simulink model "simulation"  (R2019a)
settings: Solver=VariableStepAuto  StartTime=0.0  StopTime=10  RelTol=1e-3
values from neighbouring files (symbols this model uses):
  kt = sqrt(4 * ky)    [Parameters.m]
  kx = 50    [Parameters.m]
  ky = 16 / Distance^2    (= 0.04)    [Parameters.m]
libraries: simulink x5, dspsrcs4 x1
settings Model: Creator=robot  LastModifiedBy=robot
settings DebuggingCC: AlgebraicLoopMsg=none

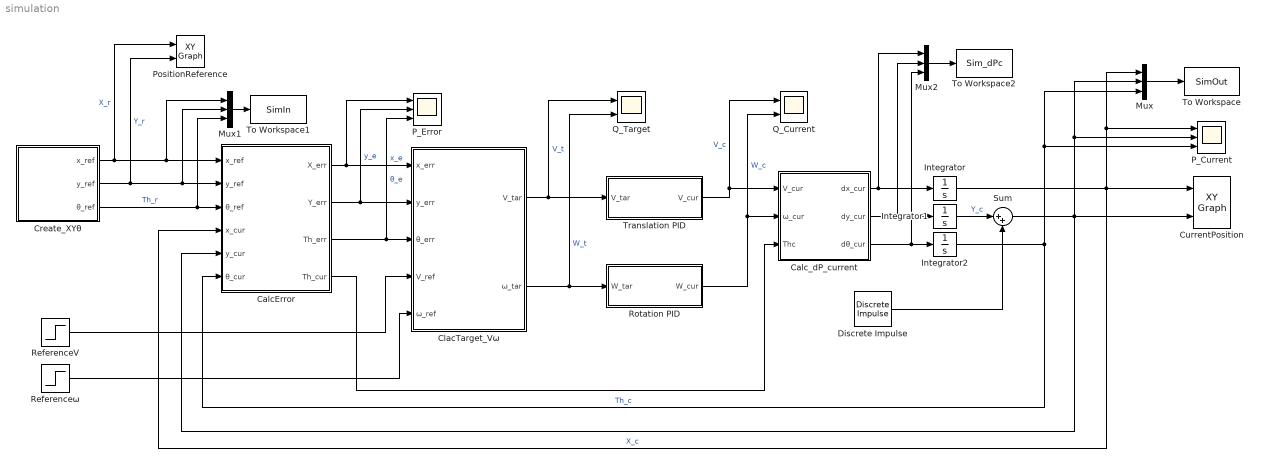
== system simulation ==
  CalcError : Subsystem
  Calc_dP_current : Subsystem
  ClacTarget_Vω : Subsystem
  Create_XYθ : Subsystem
  CurrentPosition : simulink/Sinks/XY Graph  xmin=0  xmax=200  ymin=-1  ymax=11  st=-1
  Discrete Impulse : dspsrcs4/Discrete  Impulse  Delay=6  SampleTime=1  FrameSample=1  OutputFrames=off  dataType=double  isSigned=on  wordLen=16  udDataType=sfix(16)  fracBitsMode=Best precision  numFracBits=15  OutDataTypeStr=double  LastOutDataTypeStr=double
  Integrator : Integrator
  Integrator1 : Integrator
  Integrator2 : Integrator
  Mux : Mux  Inputs=3
  Mux1 : Mux  Inputs=3
  Mux2 : Mux  Inputs=3
  P_Current : Scope  NumInputPorts=3
  P_Error : Scope  NumInputPorts=3
  PositionReference : simulink/Sinks/XY Graph  xmin=0  xmax=200  ymin=-1  ymax=11  st=-1
  Q_Current : Scope  NumInputPorts=2
  Q_Target : Scope  NumInputPorts=2
  ReferenceV : Step  Time=0  After=50  SampleTime=0.001
  Referenceω : Step  Time=0  After=0  SampleTime=0.001
  Rotation PID : Subsystem
  Sum : Sum  Inputs=|++
  To Workspace : ToWorkspace  VariableName=SimOut  SampleTime=-1
  To Workspace1 : ToWorkspace  VariableName=SimIn  SampleTime=-1
  To Workspace2 : ToWorkspace  VariableName=Sim_dPc  SampleTime=-1
  Translation PID : Subsystem
  wires:
  Create_XYθ/3(θ_ref) -> Mux1/3, CalcError/3(θ_ref)  "Th_r"
  CalcError/1(X_err) -> P_Error/1, ClacTarget_Vω/1(x_err)  "x_e"
  CalcError/2(Y_err) -> ClacTarget_Vω/2(y_err), P_Error/2  "y_e"
  CalcError/3(Th_err) -> P_Error/3, ClacTarget_Vω/3(θ_err)  "θ_e"
  ReferenceV/1 -> ClacTarget_Vω/4(V_ref)
  Referenceω/1 -> ClacTarget_Vω/5(ω_ref)
  Create_XYθ/2(y_ref) -> CalcError/2(y_ref), Mux1/2, PositionReference/2  "Y_r"
  Create_XYθ/1(x_ref) -> PositionReference/1, CalcError/1(x_ref), Mux1/1  "X_r"
  ClacTarget_Vω/1(V_tar) -> Q_Target/1, Translation PID/1(V_tar)  "V_t"
  ClacTarget_Vω/2(ω_tar) -> Q_Target/2, Rotation PID/1(W_tar)  "W_t"
  CalcError/4(Th_cur) -> Calc_dP_current/3(Thc)
  Mux/1 -> To Workspace/1
  Mux1/1 -> To Workspace1/1
  Translation PID/1(V_cur) -> Q_Current/1, Calc_dP_current/1(V_cur)  "V_c"
  Rotation PID/1(W_cur) -> Q_Current/2, Calc_dP_current/2(ω_cur)  "W_c"
  Integrator/1 -> CalcError/4(x_cur), CurrentPosition/1, Mux/1, P_Current/1  "X_c"
  Integrator1/1 -> Sum/1  "Y_c"
  Integrator2/1 -> CalcError/6(θ_cur), Mux/3, P_Current/3  "Th_c"
  Calc_dP_current/1(dx_cur) -> Mux2/1, Integrator/1
  Calc_dP_current/3(dθ_cur) -> Mux2/3, Integrator2/1
  Mux2/1 -> To Workspace2/1
  Calc_dP_current/2(dy_cur) -> Mux2/2, Integrator1/1
  Discrete Impulse/1 -> Sum/2
  Sum/1 -> CalcError/5(y_cur), Mux/2, P_Current/2, CurrentPosition/2

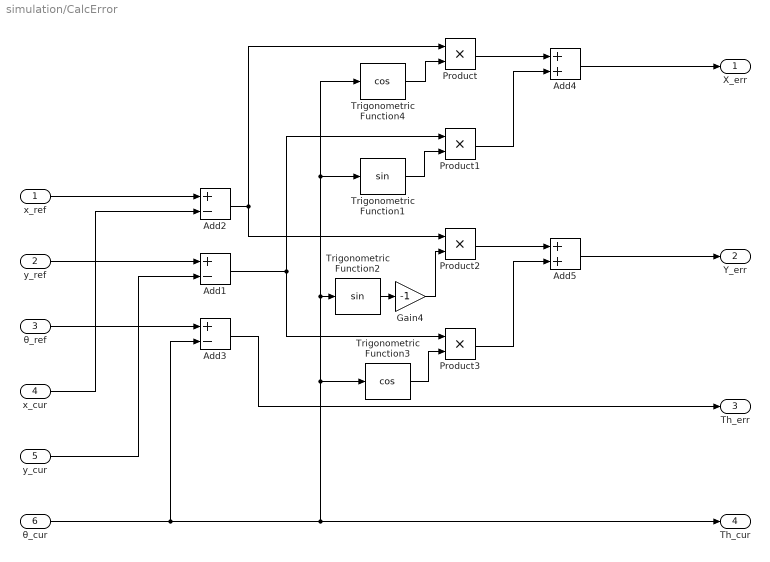
== system simulation/CalcError ==
  x_ref : Inport
  y_ref : Inport  Port=2
  θ_ref : Inport  Port=3
  x_cur : Inport  Port=4
  y_cur : Inport  Port=5
  θ_cur : Inport  Port=6
  Add1 : Sum  Inputs=+-
  Add2 : Sum  Inputs=+-
  Add3 : Sum  Inputs=+-
  Add4 : Sum
  Add5 : Sum
  Gain4 : Gain  Gain=-1
  Product{,1..3} (4 alike) : Product
  Trigonometric Function1 : Trigonometry
  Trigonometric Function2 : Trigonometry
  Trigonometric Function3 : Trigonometry  Operator=cos
  Trigonometric Function4 : Trigonometry  Operator=cos
  X_err : Outport
  Y_err : Outport  Port=2
  Th_err : Outport  Port=3
  Th_cur : Outport  Port=4
  wires:
  x_cur/1 -> Add2/2
  x_ref/1 -> Add2/1
  y_ref/1 -> Add1/1
  y_cur/1 -> Add1/2
  θ_ref/1 -> Add3/1
  θ_cur/1 -> Th_cur/1, Trigonometric Function4/1, Trigonometric Function1/1, Trigonometric Function2/1, Trigonometric Function3/1, Add3/2
  Trigonometric Function4/1 -> Product/2
  Product/1 -> Add4/1
  Trigonometric Function1/1 -> Product1/2
  Add1/1 -> Product3/1, Product1/1
  Product1/1 -> Add4/2
  Add4/1 -> X_err/1
  Add3/1 -> Th_err/1
  Add2/1 -> Product2/1, Product/1
  Product2/1 -> Add5/1
  Trigonometric Function3/1 -> Product3/2
  Product3/1 -> Add5/2
  Add5/1 -> Y_err/1
  Trigonometric Function2/1 -> Gain4/1
  Gain4/1 -> Product2/2

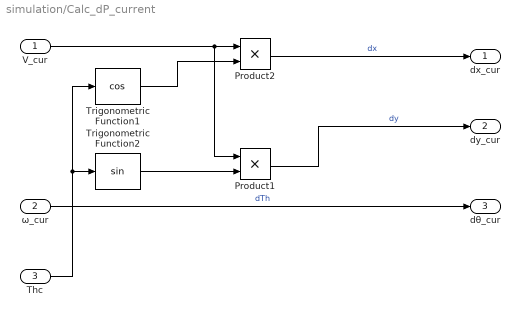
== system simulation/Calc_dP_current ==
  V_cur : Inport
  ω_cur : Inport  Port=2
  Thc : Inport  Port=3
  Product1 : Product
  Product2 : Product
  Trigonometric Function1 : Trigonometry  Operator=cos
  Trigonometric Function2 : Trigonometry
  dx_cur : Outport
  dy_cur : Outport  Port=2
  dθ_cur : Outport  Port=3
  wires:
  V_cur/1 -> Product2/1, Product1/1
  Trigonometric Function1/1 -> Product2/2
  Thc/1 -> Trigonometric Function2/1, Trigonometric Function1/1
  Product2/1 -> dx_cur/1  "dx"
  Product1/1 -> dy_cur/1  "dy"
  Trigonometric Function2/1 -> Product1/2
  ω_cur/1 -> dθ_cur/1  "dTh"

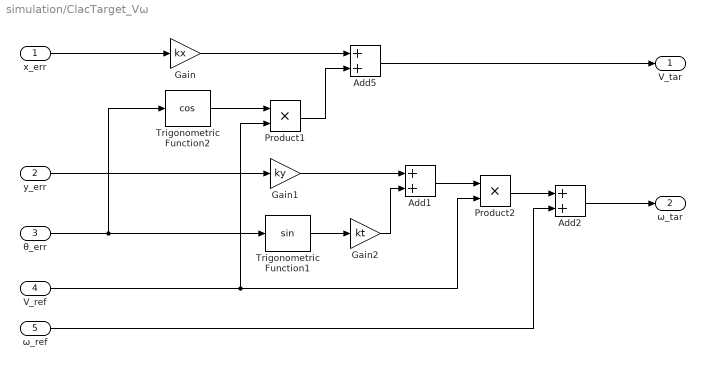
== system simulation/ClacTarget_Vω ==
  x_err : Inport
  y_err : Inport  Port=2
  θ_err : Inport  Port=3
  V_ref : Inport  Port=4
  ω_ref : Inport  Port=5
  Add1 : Sum
  Add2 : Sum
  Add5 : Sum
  Gain : Gain  Gain=kx
  Gain1 : Gain  Gain=ky
  Gain2 : Gain  Gain=kt
  Product1 : Product
  Product2 : Product
  Trigonometric Function1 : Trigonometry
  Trigonometric Function2 : Trigonometry  Operator=cos
  V_tar : Outport
  ω_tar : Outport  Port=2
  wires:
  x_err/1 -> Gain/1
  Gain/1 -> Add5/1
  θ_err/1 -> Trigonometric Function1/1, Trigonometric Function2/1
  Trigonometric Function2/1 -> Product1/1
  V_ref/1 -> Product2/2, Product1/2
  Product1/1 -> Add5/2
  Add5/1 -> V_tar/1
  y_err/1 -> Gain1/1
  Gain1/1 -> Add1/1
  Trigonometric Function1/1 -> Gain2/1
  Gain2/1 -> Add1/2
  Add1/1 -> Product2/1
  Product2/1 -> Add2/1
  ω_ref/1 -> Add2/2
  Add2/1 -> ω_tar/1

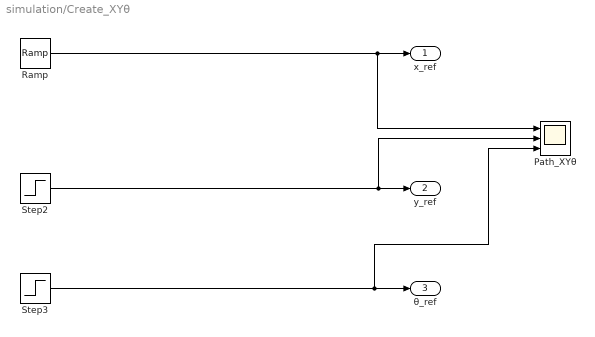
== system simulation/Create_XYθ ==
  Path_XYθ : Scope  NumInputPorts=3
  Ramp : simulink/Sources/Ramp  slope=20  start=0  InitialOutput=0
  Step2 : Step  Time=2  After=10  SampleTime=0.001
  Step3 : Step  Time=0  After=0  SampleTime=0.001
  x_ref : Outport
  y_ref : Outport  Port=2
  θ_ref : Outport  Port=3
  wires:
  Step2/1 -> Path_XYθ/2, y_ref/1
  Step3/1 -> Path_XYθ/3, θ_ref/1
  Ramp/1 -> Path_XYθ/1, x_ref/1

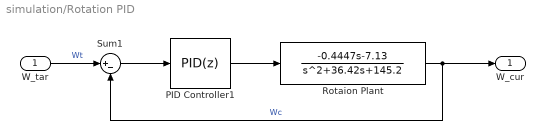
== system simulation/Rotation PID ==
  W_tar : Inport
  PID Controller1 : simulink/Continuous/PID Controller  Controller=PID  Form=Parallel  TimeDomain=Discrete-time  SampleTime=0.001  IntegratorMethod=Forward Euler  FilterMethod=Forward Euler  ControllerParametersSource=internal  P=-218.8515  I=-4309.9877  D=0  UseFilter=on  N=100  TunerSelectOption=Transfer Function Based (PID Tuner App)  InitialConditionSource=internal  InitialConditionForIntegrator=0  InitialConditionForFilter=0  DifferentiatorICPrevScaledInput=0  ExternalReset=none  TrackingMode=off  Kt=1  LimitOutput=on  UpperSaturationLimit=1200  LowerSaturationLimit=-1200  LinearizeAsGain=on  AntiWindupMode=none  Kb=1  POutMin=[]  POutMax=[]  IOutMin=[]  IOutMax=[]  DOutMin=[]  DOutMax=[]  NOutMin=[]  NOutMax=[]  SumOutMin=[]  SumOutMax=[]  SaturationOutMin=[]  SaturationOutMax=[]  PParamMin=[]  PParamMax=[]  IParamMin=[]  IParamMax=[]  DParamMin=[]  DParamMax=[]  NParamMin=[]  NParamMax=[]  KbParamMin=[]  KbParamMax=[]  KtParamMin=[]  KtParamMax=[]  KbOutMin=[]  KbOutMax=[]  KtOutMin=[]  KtOutMax=[]  IntegratorOutMin=[]  IntegratorOutMax=[]  FilterOutMin=[]  FilterOutMax=[]  SumI1OutMin=[]  SumI1OutMax=[]  SumI2OutMin=[]  SumI2OutMax=[]  SumI3OutMin=[]  SumI3OutMax=[]  SumI4OutMin=[]  SumI4OutMax=[]  SumDOutMin=[]  SumDOutMax=[]  DifferentiatorOutMin=[]  DifferentiatorOutMax=[]  FilterDiffOutCoefMin=[]  FilterDiffOutCoefMax=[]  ReciprocalOutMin=[]  ReciprocalOutMax=[]  SumDenOutMin=[]  SumDenOutMax=[]  SumNumOutMin=[]  SumNumOutMax=[]  DivideOutMin=[]  DivideOutMax=[]  IntegratorContinuousStateAttributes=''  IntegratorStateMustResolveToSignalObject=off  IntegratorRTWStateStorageClass=Auto  FilterContinuousStateAttributes=''  FilterStateMustResolveToSignalObject=off  FilterRTWStateStorageClass=Auto  ParallelPVariant=InternalParameters  IdealPVariant=Disabled  IVariant=InternalParameters  DVariant=InternalParameters  IntegratorVariant=Discrete  SatVariant=Enabled  AWVariant=Passthrough  PCopyVariant=Disabled  TRVariant=Disabled  FdbkBlocksVariant=Forward  IdealPFdbkVariant=Disabled  SatFdbkVariant=Disabled  DerivativeFilterVariant=ForwardEulerFilter  NVariant=InternalParameters  NCopyVariant=Disabled  FilterICVariant=InternalICsFilter  IntegratorICVariant=InternalICs  ExternalResetVariant=Disabled  TRSumVariant=Passthrough  SumFdbkVariant=Disabled  SumVariant=Sum_PID
  Rotaion Plant : TransferFcn  Numerator=[-0.4447 -7.13]  Denominator=[1 36.42 145.2]
  Sum1 : Sum  Inputs=|+-
  W_cur : Outport
  wires:
  PID Controller1/1 -> Rotaion Plant/1
  Sum1/1 -> PID Controller1/1
  W_tar/1 -> Sum1/1  "Wt"
  Rotaion Plant/1 -> Sum1/2, W_cur/1  "Wc"

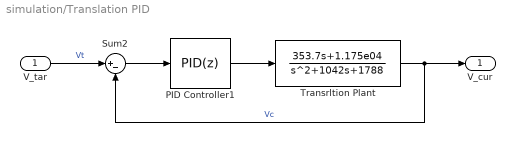
== system simulation/Translation PID ==
  V_tar : Inport
  PID Controller1 : simulink/Continuous/PID Controller  Controller=PID  Form=Parallel  TimeDomain=Discrete-time  SampleTime=0.001  IntegratorMethod=Forward Euler  FilterMethod=Forward Euler  ControllerParametersSource=internal  P=0.73598  I=3.7518  D=0  UseFilter=on  N=100  TunerSelectOption=Transfer Function Based (PID Tuner App)  InitialConditionSource=internal  InitialConditionForIntegrator=0  InitialConditionForFilter=0  DifferentiatorICPrevScaledInput=0  ExternalReset=none  TrackingMode=off  Kt=1  LimitOutput=on  UpperSaturationLimit=1200  LowerSaturationLimit=-1200  LinearizeAsGain=on  AntiWindupMode=none  Kb=1  POutMin=[]  POutMax=[]  IOutMin=[]  IOutMax=[]  DOutMin=[]  DOutMax=[]  NOutMin=[]  NOutMax=[]  SumOutMin=[]  SumOutMax=[]  SaturationOutMin=[]  SaturationOutMax=[]  PParamMin=[]  PParamMax=[]  IParamMin=[]  IParamMax=[]  DParamMin=[]  DParamMax=[]  NParamMin=[]  NParamMax=[]  KbParamMin=[]  KbParamMax=[]  KtParamMin=[]  KtParamMax=[]  KbOutMin=[]  KbOutMax=[]  KtOutMin=[]  KtOutMax=[]  IntegratorOutMin=[]  IntegratorOutMax=[]  FilterOutMin=[]  FilterOutMax=[]  SumI1OutMin=[]  SumI1OutMax=[]  SumI2OutMin=[]  SumI2OutMax=[]  SumI3OutMin=[]  SumI3OutMax=[]  SumI4OutMin=[]  SumI4OutMax=[]  SumDOutMin=[]  SumDOutMax=[]  DifferentiatorOutMin=[]  DifferentiatorOutMax=[]  FilterDiffOutCoefMin=[]  FilterDiffOutCoefMax=[]  ReciprocalOutMin=[]  ReciprocalOutMax=[]  SumDenOutMin=[]  SumDenOutMax=[]  SumNumOutMin=[]  SumNumOutMax=[]  DivideOutMin=[]  DivideOutMax=[]  IntegratorContinuousStateAttributes=''  IntegratorStateMustResolveToSignalObject=off  IntegratorRTWStateStorageClass=Auto  FilterContinuousStateAttributes=''  FilterStateMustResolveToSignalObject=off  FilterRTWStateStorageClass=Auto  ParallelPVariant=InternalParameters  IdealPVariant=Disabled  IVariant=InternalParameters  DVariant=InternalParameters  IntegratorVariant=Discrete  SatVariant=Enabled  AWVariant=Passthrough  PCopyVariant=Disabled  TRVariant=Disabled  FdbkBlocksVariant=Forward  IdealPFdbkVariant=Disabled  SatFdbkVariant=Disabled  DerivativeFilterVariant=ForwardEulerFilter  NVariant=InternalParameters  NCopyVariant=Disabled  FilterICVariant=InternalICsFilter  IntegratorICVariant=InternalICs  ExternalResetVariant=Disabled  TRSumVariant=Passthrough  SumFdbkVariant=Disabled  SumVariant=Sum_PID
  Sum2 : Sum  Inputs=|+-
  Transrltion Plant : TransferFcn  Numerator=[353.7 1.175e04]  Denominator=[1 1042 1788]
  V_cur : Outport
  wires:
  Sum2/1 -> PID Controller1/1
  PID Controller1/1 -> Transrltion Plant/1
  Transrltion Plant/1 -> V_cur/1, Sum2/2  "Vc"
  V_tar/1 -> Sum2/1  "Vt"
